simulink model "px4_sendQuat"  (R2018b)
settings: Solver=FixedStepAuto  StartTime=0.0  StopTime=inf  RelTol=1e-3  EnableMultiTasking=on
libraries: px4lib x1, px4Sensorslib x1
settings Model: SimulationMode=external  ExtModeTrigDuration=10  Creator=Robert  LastModifiedBy=Robert
settings SolverCC: PositivePriorityOrder=on
settings OptimizationCC: EnhancedBackFolding=on  PassReuseOutputArgsAs=Individual arguments  MaxStackSize=64  OptimizeBlockOrder=speed  DifferentSizesBufferReuse=on  OptimizationCustomize=off
settings DebuggingCC: ParameterTunabilityLossMsg=error
settings HardwareCC: ProdBitPerPointer=32  ProdBitPerSizeT=32  ProdBitPerPtrDiffT=32  ProdLargestAtomicInteger=Long  ProdLargestAtomicFloat=Double  ProdWordSize=32  ProdLongLongMode=on  ProdHWDeviceType=ARM Compatible->ARM Cortex
settings SFSimCC: MATLABDynamicMemAlloc=off
settings RTWCC: SystemTargetFile=ert.tlc  HardwareBoard=PX4 Pixhawk 1  TLCOptions="-aInlineSetEventsForThisBaseRateFcn=TLC_FALSE -aSuppressMultiTaskScheduler=TLC_FALSE  -aRateBasedStepFcn=0"  TemplateMakefile=ert_default_tmf  GenerateReport=on  Toolchain=GNU Tools for PX4 Autopilots  IncludeHyperlinkInReport=on  LaunchReport=on  TargetLang=C++  GenerateTraceInfo=on  GenerateTraceReport=on  GenerateTraceReportSl=on  GenerateTraceReportSf=on  GenerateTraceReportEml=on
settings CodeAppCC: ForceParamTrailComments=on  IgnoreCustomStorageClasses=off  OperatorAnnotations=on  SimulinkDataObjDesc=on  SFDataObjDesc=on  InsertBlockDesc=on

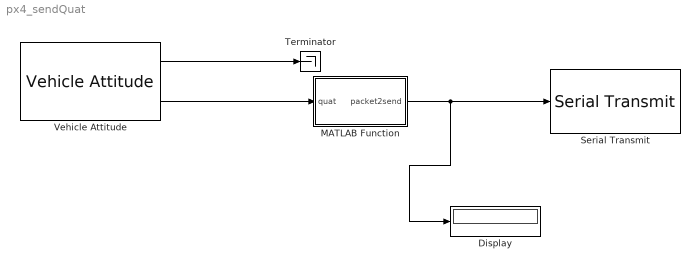
== system px4_sendQuat ==
  Display : Display
  MATLAB Function : MATLAB Function  TreatAsAtomicUnit=on
  Serial Transmit : px4lib/Serial Transmit  SCIModule=/dev/ttyACM0
      settings: SourceProductName=Embedded Coder Support Package for PX4 Autopilots  SourceProductBaseCode=PX4AUTOPILOTS
  Terminator : Terminator
  Vehicle Attitude : px4Sensorslib/Vehicle Attitude  rollRate=off  pitchRate=off  yawRate=off  quaternion=on  uorbTimeStamp=off  BlockingMode=off  BlockTimeout=0.001  sampleTime=0.01
      settings: SourceProductName=Embedded Coder Support Package for PX4 Autopilots
  wires:
  Vehicle Attitude/2 -> MATLAB Function/1(quat)
  MATLAB Function/1(packet2send) -> Display/1, Serial Transmit/1
  Vehicle Attitude/1 -> Terminator/1

== matlab function px4_sendQuat/MATLAB Function ==
  data: quat input; packet2send output
function packet2send = packetquat(quat)
packet2send = uint8(zeros(1,17));

header = uint8('A');
%footer = uint8('B');

q = typecast(single(quat),'uint8');
%q = typecast(single([1.1 2.2 3.3 4.4]),'uint8');
packet2send = [header q];% footer];
%packet2send = [uint8(0) single(1) single(2) single(3) single(4) uint8(5)];
